simulink model "kalman_vel_est"  (R2022a)
settings: Solver=VariableStepAuto  StartTime=0.0  StopTime=20  RelTol=1e-3
values from neighbouring files (symbols this model uses):
  A = [0 1 0 0 0; 0 0 0 0 0; 0 0 0 1 0; 0 0 0 0 1; 0 0 0 0 0]    [Kalman_vel_est.m]    (also in continues_time_state_space.m = [0 1 0 0; 0 0 0 0; 0 0 0 omega; 0 0 -omega 0])
  B = [0; 1; 0; 0; 0]    [Kalman_vel_est.m]
  C = [1 0 -1 0 0; 1 0 0 0 0]    [Kalman_vel_est.m]
  dt = 0.1    [Kalman_vel_est.m]    (also in UKF_test.m; state_transfer.m = 0.02; states.m)
  R = [1 0; 0 1]    [Kalman_vel_est.m]
  sys_d = c2d(sys,dt)    [Kalman_vel_est.m]
  x0 = [10 0 0 1 0]    [Kalman_vel_est.m]
undefined symbols (not defined in the file or in its folder): Continuous, Discrete, Time
libraries: simulink x4, ctrlSharedLib x2
settings Model: Creator=Bruger  LastModifiedBy=soren
settings SolverCC: AlgebraicLoopSolver=TrustRegion
settings DebuggingCC: UnconnectedInputMsg=warning  UnconnectedOutputMsg=warning  UnconnectedLineMsg=warning  SFMachineParentedDataDiag=warning
settings RTWCC: DLArmComputeVersion=19.05

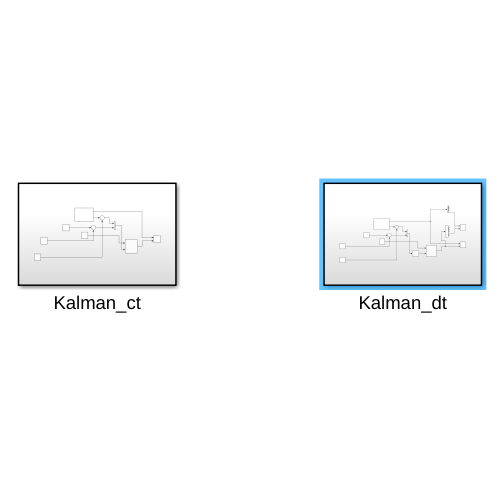
[thumbnail: Simulink's stored preview of the top-level diagram]
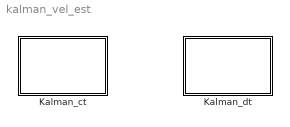
== system kalman_vel_est ==
  Kalman_ct : Subsystem
  Kalman_dt : Subsystem

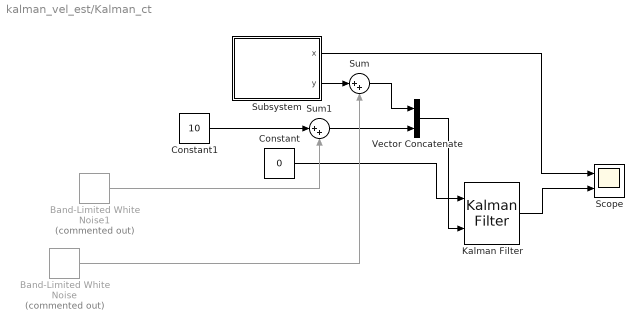
== system kalman_vel_est/Kalman_ct ==
  Band-Limited White Noise : simulink/Sources/Band-Limited White Noise  Commented=on  Cov=[1]  Ts=0.1  seed=[23341]
  Band-Limited White Noise1 : simulink/Sources/Band-Limited White Noise  Commented=on  Cov=[1]  Ts=0.1  seed=[23341]
  Constant : Constant  Value=0
  Constant1 : Constant  Value=10
  Kalman Filter : ctrlSharedLib/Kalman Filter  TimeDomain=Continuous-Time  UseCurrentEstimator=on  ModelSource=Individual A, B, C, D matrices  ModelSourceVariable=ss(0.95,1,1,0,1)  A=A  B=B  C=C  D=0  NumberOfStates=1  NumberOfInputs=1  NumberOfOutputs=1  InitialEstimateSource=Dialog  X0=x0  P0=10  UseK=off  UseGH=off  NumberOfProcessNoiseInputs=1  G=1  TimeInvariantG=on  H=0  TimeInvariantH=on  Q=Q  TimeInvariantQ=on  R=R  TimeInvariantR=on  N=0  TimeInvariantN=on  AddInputPort=on  AddEnablePort=off  OutputEstimatedY=off  OutputP=off  Ts=-1
  Scope : Scope  NumInputPorts=2
  Subsystem : Subsystem
  Sum : Sum  Inputs=|++
  Sum1 : Sum  Inputs=|++
  Vector Concatenate : Concatenate
  wires:
  Subsystem/2(y) -> Sum/1
  Sum1/1 -> Vector Concatenate/2
  Sum/1 -> Vector Concatenate/1
  Constant/1 -> Kalman Filter/1
  Kalman Filter/1 -> Scope/2
  Band-Limited White Noise1/1 -> Sum1/2
  Constant1/1 -> Sum1/1
  Subsystem/1(x) -> Scope/1
  Vector Concatenate/1 -> Kalman Filter/2
  Band-Limited White Noise/1 -> Sum/2

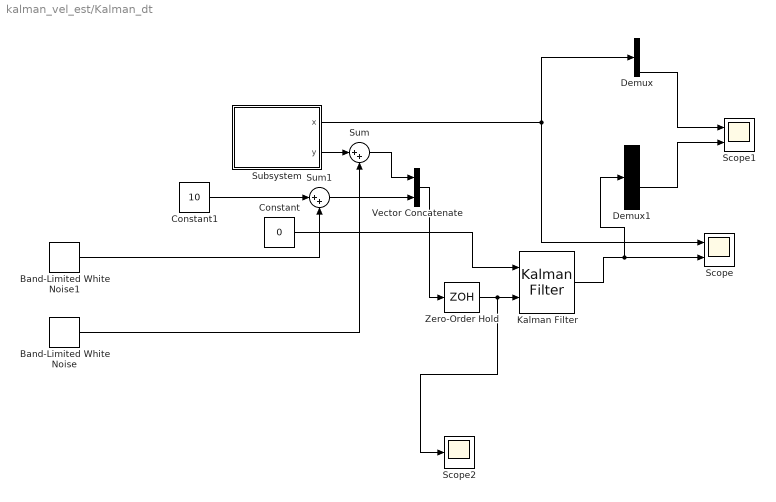
== system kalman_vel_est/Kalman_dt ==
  Band-Limited White Noise : simulink/Sources/Band-Limited White Noise  Cov=[0.0001]  Ts=0.1  seed=[23321]
  Band-Limited White Noise1 : simulink/Sources/Band-Limited White Noise  Cov=[0.0001]  Ts=0.1  seed=[23341]
  Constant : Constant  Value=0
  Constant1 : Constant  Value=10
  Demux : Demux
  Demux1 : Demux  Outputs=5
  Kalman Filter : ctrlSharedLib/Kalman Filter  TimeDomain=Discrete-Time  UseCurrentEstimator=on  ModelSource=Individual A, B, C, D matrices  ModelSourceVariable=ss(0.95,1,1,0,1)  A=sys_d.A  B=sys_d.B  C=sys_d.C  D=0  NumberOfStates=1  NumberOfInputs=1  NumberOfOutputs=1  InitialEstimateSource=Dialog  X0=x0  P0=10  UseK=off  UseGH=off  NumberOfProcessNoiseInputs=1  G=1  TimeInvariantG=on  H=0  TimeInvariantH=on  Q=Q  TimeInvariantQ=on  R=R  TimeInvariantR=on  N=0  TimeInvariantN=on  AddInputPort=on  AddEnablePort=off  OutputEstimatedY=off  OutputP=off  Ts=dt
  Scope : Scope  NumInputPorts=2
  Scope1 : Scope  NumInputPorts=2
  Scope2 : Scope
  Subsystem : Subsystem
  Sum : Sum  Inputs=|++
  Sum1 : Sum  Inputs=|++
  Vector Concatenate : Concatenate
  Zero-Order Hold : ZeroOrderHold  SampleTime=dt
  wires:
  Subsystem/2(y) -> Sum/1
  Sum1/1 -> Vector Concatenate/2
  Sum/1 -> Vector Concatenate/1
  Constant/1 -> Kalman Filter/1
  Kalman Filter/1 -> Demux1/1, Scope/2
  Band-Limited White Noise1/1 -> Sum1/2
  Constant1/1 -> Sum1/1
  Subsystem/1(x) -> Scope/1, Demux/1
  Band-Limited White Noise/1 -> Sum/2
  Vector Concatenate/1 -> Zero-Order Hold/1
  Zero-Order Hold/1 -> Scope2/1, Kalman Filter/2
  Demux/4 -> Scope1/1
  Demux1/4 -> Scope1/2

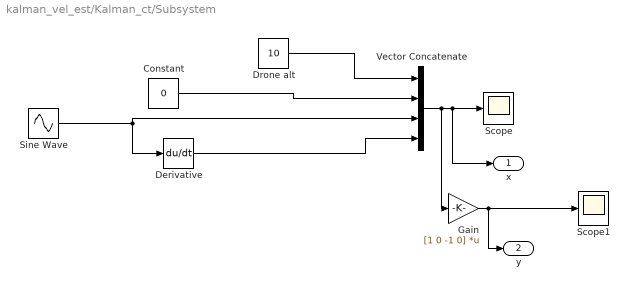
== system kalman_vel_est/Kalman_ct/Subsystem ==
  Constant : Constant  Value=0
  Derivative : Derivative
  Drone alt : Constant  Value=10
  Gain : Gain  Gain=[1 0 -1 0]  Multiplication=Matrix(K*u) (u vector)
  Scope : Scope
  Scope1 : Scope
  Sine Wave : Sin  SampleTime=0
  Vector Concatenate : Concatenate  NumInputs=4
  x : Outport
  y : Outport  Port=2
  wires:
  Constant/1 -> Vector Concatenate/2
  Vector Concatenate/1 -> Gain/1, x/1, Scope/1
  Derivative/1 -> Vector Concatenate/4
  Sine Wave/1 -> Derivative/1, Vector Concatenate/3
  Drone alt/1 -> Vector Concatenate/1
  Gain/1 -> y/1, Scope1/1

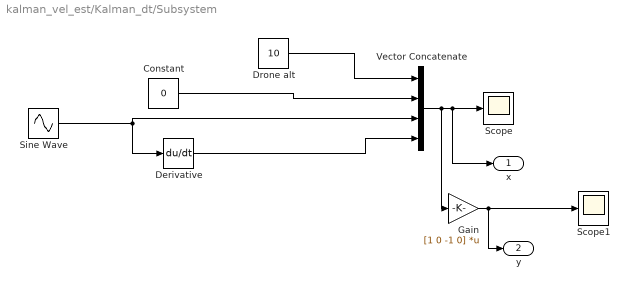
== system kalman_vel_est/Kalman_dt/Subsystem ==
  Constant : Constant  Value=0
  Derivative : Derivative
  Drone alt : Constant  Value=10
  Gain : Gain  Gain=[1 0 -1 0]  Multiplication=Matrix(K*u) (u vector)
  Scope : Scope
  Scope1 : Scope
  Sine Wave : Sin  Amplitude=0.5  SampleTime=0
  Vector Concatenate : Concatenate  NumInputs=4
  x : Outport
  y : Outport  Port=2
  wires:
  Constant/1 -> Vector Concatenate/2
  Vector Concatenate/1 -> Gain/1, x/1, Scope/1
  Derivative/1 -> Vector Concatenate/4
  Sine Wave/1 -> Derivative/1, Vector Concatenate/3
  Drone alt/1 -> Vector Concatenate/1
  Gain/1 -> y/1, Scope1/1
